simulink model "hdlcoderdft_testbench"  (R2017a)
settings: Solver=FixedStepDiscrete  StartTime=0.0  StopTime=analysisDuration  FixedStep=sampleTime  RelTol=1e-3
PostLoadFcn:
  | hdlcoderdft_testbench_init
InitFcn:
  | hdlcoderdft_testbench_init
values from neighbouring files (symbols this model uses):
  nDistances = 4    [hdlcoderdft_init.m]
  nFilters = 4    [hdlcoderdft_init.m]
  nRecurrences = 4    [hdlcoderdft_testbench_init.m]
  recurrencePeriod = sampleTime * nDistances    [hdlcoderdft_testbench_init.m]
  sampleFrequency = 150 * MHz    (= 150000000)    [hdlcoderdft_testbench_init.m]
  sampleTime = 1.0 / sampleFrequency    (= 6.66666666667e-09)    [hdlcoderdft_testbench_init.m]
  startFilter = 0    [hdlcoderdft_testbench_init.m]
settings Model: DataTypeOverride=Off  Creator=Pierre BERNARDI  LastModifiedBy=Pierre BERNARDI
settings DataIOCC: LimitDataPoints=on  SaveOutput=off  SaveTime=off
settings OptimizationCC: BlockReduction=off  ConditionallyExecuteInputs=off  DefaultParameterBehavior=Inlined  LifeSpan=inf
settings DebuggingCC: AlgebraicLoopMsg=error  SingleTaskRateTransMsg=error  AllowSymbolicDim=off  StrictBusMsg=ErrorOnBusTreatedAsVector  SFUnexpectedBacktrackingDiag=warning  SFNoUnconditionalDefaultTransitionDiag=warning  SFExecutionAtInitializationDiag=none
settings HardwareCC: ProdBitPerPointer=32  ProdBitPerSizeT=32  ProdBitPerPtrDiffT=32  ProdLargestAtomicFloat=None  ProdIntDivRoundTo=Undefined  ProdEndianess=Unspecified  ProdWordSize=32  ProdHWDeviceType=ASIC/FPGA->ASIC/FPGA  ProdEqTarget=off
settings GRTTargetCC: TargetLangStandard=C89/C90 (ANSI)  GeneratePreprocessorConditionals=Disable all
settings ConfigComp: CovScope=ReferencedModels  CovMetricSettings=dw  CovHtmlReporting=on  CovSaveCumulativeToWorkspaceVar=on  CovSaveSingleToWorkspaceVar=on  CovExternalEMLEnable=off  CovSFcnEnable=off

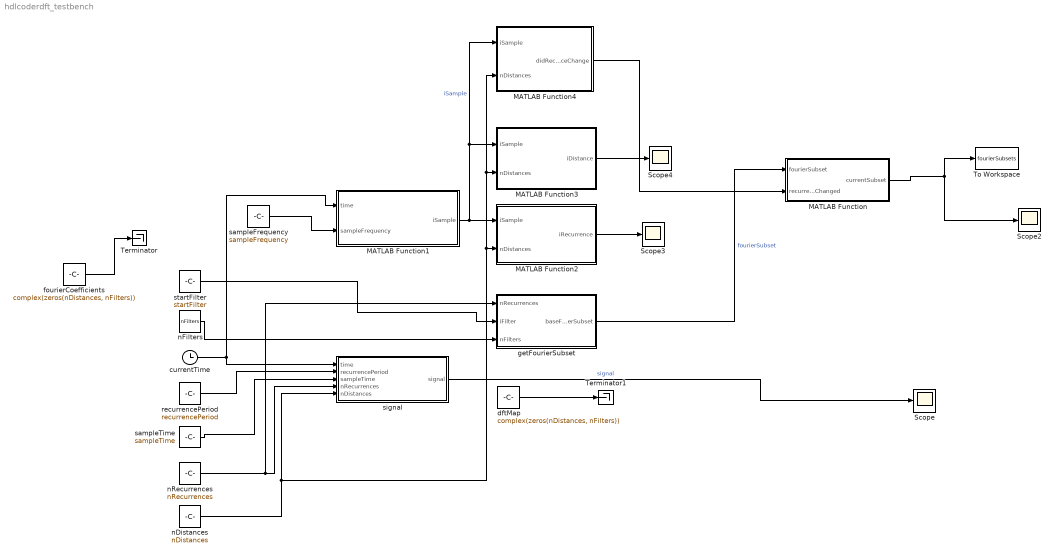
== system hdlcoderdft_testbench ==
  MATLAB Function : MATLAB Function  TreatAsAtomicUnit=on
  MATLAB Function1 : MATLAB Function  TreatAsAtomicUnit=on
  MATLAB Function2 : MATLAB Function  TreatAsAtomicUnit=on
  MATLAB Function3 : MATLAB Function  TreatAsAtomicUnit=on
  MATLAB Function4 : MATLAB Function  TreatAsAtomicUnit=on
  Scope{,2..4} (4 alike) : Scope
  Terminator : Terminator
  Terminator1 : Terminator
  To Workspace : ToWorkspace  VariableName=fourierSubsets  SaveFormat=Structure With Time  SampleTime=-1
  currentTime : Clock
  dftMap : Constant  Value=complex(zeros(nDistances, nFilters))
  fourierCoefficients : Constant  Value=complex(zeros(nDistances, nFilters))  OutDataTypeStr=double
  getFourierSubset : MATLAB Function  TreatAsAtomicUnit=on
  nDistances : Constant  Value=nDistances  OutDataTypeStr=uint16
  nFilters : Constant  Value=nFilters
  nRecurrences : Constant  Value=nRecurrences  OutDataTypeStr=uint16
  recurrencePeriod : Constant  Value=recurrencePeriod  OutDataTypeStr=double
  sampleFrequency : Constant  Value=sampleFrequency
  sampleTime : Constant  Value=sampleTime  OutDataTypeStr=double
  signal : MATLAB Function  TreatAsAtomicUnit=on
  startFilter : Constant  Value=startFilter
  wires:
  recurrencePeriod/1 -> signal/2(recurrencePeriod)
  nRecurrences/1 -> getFourierSubset/1(nRecurrences), signal/4(nRecurrences)
  currentTime/1 -> MATLAB Function1/1(time), signal/1(time)
  sampleTime/1 -> signal/3(sampleTime)
  signal/1(signal) -> Scope/1  "signal"
  nFilters/1 -> getFourierSubset/3(nFilters)
  startFilter/1 -> getFourierSubset/2(iFilter)
  fourierCoefficients/1 -> Terminator/1
  getFourierSubset/1(baseFourierSubset) -> MATLAB Function/1(fourierSubset)  "fourierSubset"
  MATLAB Function/1(currentSubset) -> To Workspace/1, Scope2/1
  sampleFrequency/1 -> MATLAB Function1/2(sampleFrequency)
  MATLAB Function1/1(iSample) -> MATLAB Function3/1(iSample), MATLAB Function4/1(iSample), MATLAB Function2/1(iSample)  "iSample"
  MATLAB Function2/1(iRecurrence) -> Scope3/1
  nDistances/1 -> MATLAB Function4/2(nDistances), MATLAB Function3/2(nDistances), MATLAB Function2/2(nDistances), signal/5(nDistances)
  MATLAB Function3/1(iDistance) -> Scope4/1
  dftMap/1 -> Terminator1/1
  MATLAB Function4/1(didRecurrenceChange) -> MATLAB Function/2(recurrenceChanged)

== matlab function hdlcoderdft_testbench/getFourierSubset ==
  settings: updateMethod=DISCRETE  sampleTime=sampleTime
  data: nRecurrences input size=1; baseFourierSubset output double size=[nFilters 1]; iFilter input size=1; nFilters input size=1
function baseFourierSubset = baseFourierSubset(nRecurrences, iFilter, nFilters)
    persistent fourierSubset
    if(isempty(fourierSubset))
        fourierSubset = getBaseFourierSubset(double(nRecurrences), iFilter, nFilters)
    end
    baseFourierSubset = fourierSubset
end

== matlab function hdlcoderdft_testbench/signal ==
  settings: updateMethod=DISCRETE  sampleTime=sampleTime
  data: time input double; signal output double size=1; recurrencePeriod input double size=1; sampleTime input double size=1; nRecurrences input uint16 size=1; nDistances input uint16 size=1
function signal = signal(time, recurrencePeriod, sampleTime, nRecurrences, nDistances)
    iRecurrence = double(getRecurrenceId(time, recurrencePeriod))
    iDoor       = double(getDoorId(time, sampleTime, recurrencePeriod, nDistances))
    signal      = complex(exp(2j * pi * iRecurrence * iDoor / double(nRecurrences)))
end

== matlab function hdlcoderdft_testbench/MATLAB Function ==
  settings: updateMethod=DISCRETE  sampleTime=sampleTime
  data: fourierSubset input double size=[nFilters 1]; currentSubset output double size=[nFilters 1]; recurrenceChanged input boolean
function currentSubset = recursiveMultiply(fourierSubset, recurrenceChanged)
    persistent previousSubset
    if(isempty(previousSubset))
        previousSubset = conj(fourierSubset)
    end
    if recurrenceChanged
        previousSubset = previousSubset .* fourierSubset
    end
    currentSubset  = previousSubset
end

== matlab function hdlcoderdft_testbench/MATLAB Function1 ==
  data: time input double size=1; iSample output uint16 size=1; sampleFrequency input double size=1
function iSample = sampleId(time, sampleFrequency)
    iSample = uint16(getSampleId(time, sampleFrequency))
end

== matlab function hdlcoderdft_testbench/MATLAB Function2 ==
  data: iSample input uint16 size=1; iRecurrence output uint16 size=1; nDistances input uint16 size=1
function iRecurrence = recurrenceId(iSample, nDistances)
    iRecurrence = getRecurrenceId2(iSample, nDistances)
end

== matlab function hdlcoderdft_testbench/MATLAB Function3 ==
  data: iSample input uint16 size=1; iDistance output uint16 size=1; nDistances input uint16 size=1
function iDistance = distanceId(iSample, nDistances)
    iDistance = getDistanceId(iSample, nDistances)
end

== matlab function hdlcoderdft_testbench/MATLAB Function4 ==
  data: iSample input uint16 size=1; didRecurrenceChange output boolean size=1; nDistances input uint16 size=1
function didRecurrenceChange = recurrenceDidChange(iSample, nDistances)
    didRecurrenceChange = recurrenceChanged(iSample, nDistances)
end
